simulink model "DCmotormodelREF"  (R2024b)
settings: Solver=VariableStepAuto  StartTime=0.0  StopTime=18  MaxStep=1e-4  RelTol=1e-4  AbsTol=1e-5
values from neighbouring files (symbols this model uses):
  Ctot = TMa/10 + 0.072 + Jmotor * omega_max_rad/ta    (= 0.152406290556)    [DCMOTORELAST.m]    (also in simulazione_vuota1.mat = 0.152406290545; simulazione_vuota2lim.mat = 0.152406290545)
  ilim = 1*Ia_nom    (= 3.65)    [DCMOTORELAST.m]    (also in simulazione_vuota1.mat = 4.38; simulazione_vuota2lim.mat = 4.38)
  Jtot = (Ctot*ta) / omega_max_rad    (= 0.000727686435009)    [DCMOTORELAST.m]    (also in simulazione_vuota1.mat = 0.000727686435787; simulazione_vuota2lim.mat = 0.000727686435787)
  kamp = Va_lim/dcvolt    (= 5.76)    [DCMOTORELAST.m]    (also in simulazione_vuota1.mat; simulazione_vuota2lim.mat)
  kdt = Vctr/omega_max_rad    (= 0.0131293711322)    [DCMOTORELAST.m]    (also in simulazione_vuota1.mat = 0.0131278037994; simulazione_vuota2lim.mat = 0.0131278037994)
  kff = kv/(kamp*kdt)    (= 0.921781173607)    [DCMOTORELAST.m]
  ki = Ki_opt    (= 56)    [DCMOTORELAST.m]
  klim_corr = dcvolt/(0.2*Ia_nom)    (= 6.84931506849)    [DCMOTORELAST.m]    (also in simulazione_vuota1.mat; simulazione_vuota2lim.mat)
  kp = kpf    [DCMOTORELAST.m]
  Kpos = Kpos_vec(ii)    [DCMOTORELAST.m]
  kt = kv    (= 0.0697098650743)    [DCMOTORELAST.m]    (also in simulazione_vuota1.mat = 0.0697; simulazione_vuota2lim.mat = 0.0697)
  kv = kvC*60/(1000*2*pi)    (= 0.0697098650743)    [DCMOTORELAST.m]    (also in simulazione_vuota1.mat = 0.0697; simulazione_vuota2lim.mat = 0.0697)
  S_wu = 1.2*(Ra*Iamax/kamp)    (= 0.387156307417)    [DCMOTORELAST.m]
  Va_lim = 1.2*Va_nom    (= 28.8)    [DCMOTORELAST.m]    (also in simulazione_vuota1.mat; simulazione_vuota2lim.mat)
  Vctr = Va/kamp    (= 4.12471358951)    [DCMOTORELAST.m]    (also in simulazione_vuota1.mat = 4.12422119268; simulazione_vuota2lim.mat = 4.12422119268)
libraries: cstblocks x2
settings Model: Creator=marco  LastModifiedBy=david

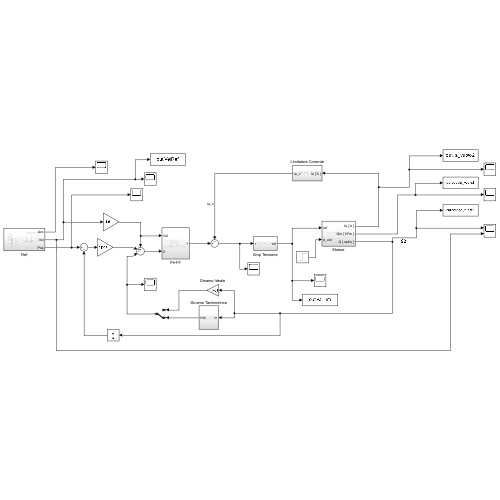
[thumbnail: Simulink's stored preview of the top-level diagram]
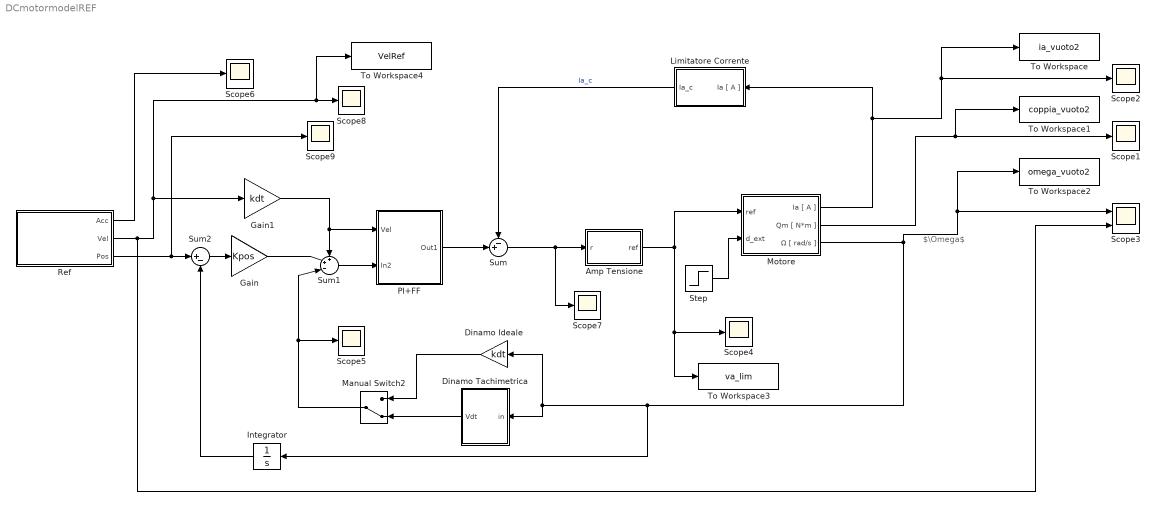
== system DCmotormodelREF ==
  note: $\Omega$
  Amp Tensione : Subsystem
  Dinamo Ideale : Gain  Gain=kdt
  Dinamo Tachimetrica : Subsystem
  Gain : Gain  Gain=Kpos
  Gain1 : Gain  Gain=kdt
  Integrator : Integrator
  Limitatore Corrente : Subsystem
  Manual Switch2 : ManualSwitch  CurrentSetting=0
  Motore : Subsystem
  PI+FF : Subsystem
  Ref : Subsystem
  Scope{1..2,4..9} (8 alike) : Scope
  Scope3 : Scope  NumInputPorts=2
  Step : Step  Time=5  After=Vctr*0.8*0.01  SampleTime=0
  Sum : Sum  Inputs=-+|
  Sum1 : Sum  Inputs=++-|
  Sum2 : Sum  Inputs=|+-
  To Workspace : ToWorkspace  VariableName=ia_vuoto2  SaveFormat=Timeseries  SampleTime=-1
  To Workspace1 : ToWorkspace  VariableName=coppia_vuoto2  SaveFormat=Timeseries  SampleTime=-1
  To Workspace2 : ToWorkspace  VariableName=omega_vuoto2  SaveFormat=Timeseries  SampleTime=-1
  To Workspace3 : ToWorkspace  VariableName=va_lim  SaveFormat=Timeseries  SampleTime=-1
  To Workspace4 : ToWorkspace  VariableName=VelRef  SaveFormat=Timeseries  SampleTime=-1
  wires:
  Motore/1(Ia [ A ]) -> Limitatore Corrente/1(Ia [ A ]), To Workspace/1, Scope2/1
  Motore/2(Qm [ N*m ]) -> To Workspace1/1, Scope1/1
  Motore/3(Ω [ rad/s ]) -> To Workspace2/1, Scope3/1, Integrator/1, Dinamo Tachimetrica/1(in), Dinamo Ideale/1
  Amp Tensione/1(ref) -> Motore/1(ref), Scope4/1, To Workspace3/1
  Sum/1 -> Amp Tensione/1(r), Scope7/1
  Limitatore Corrente/1(Ia_c) -> Sum/1  "Ia_c"
  Dinamo Tachimetrica/1(Vdt) -> Manual Switch2/2
  Manual Switch2/1 -> Scope5/1, Sum1/3
  Dinamo Ideale/1 -> Manual Switch2/1
  Sum1/1 -> PI+FF/2(In2)
  PI+FF/1(Out1) -> Sum/2
  Ref/1(Acc) -> Scope6/1
  Ref/2(Vel) -> Scope3/2, To Workspace4/1, Scope8/1, Gain1/1
  Ref/3(Pos) -> Sum2/1, Scope9/1
  Integrator/1 -> Sum2/2
  Sum2/1 -> Gain/1
  Gain/1 -> Sum1/2
  Gain1/1 -> Sum1/1, PI+FF/1(Vel)
  Step/1 -> Motore/2(d_ext)

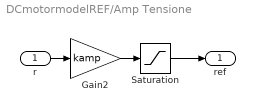
== system DCmotormodelREF/Amp Tensione ==
  r : Inport
  Gain2 : Gain  Gain=kamp
  Saturation : Saturate  UpperLimit=Va_lim  LowerLimit=-Va_lim
  ref : Outport
  wires:
  Saturation/1 -> ref/1
  Gain2/1 -> Saturation/1
  r/1 -> Gain2/1

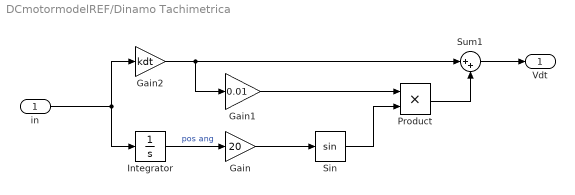
== system DCmotormodelREF/Dinamo Tachimetrica ==
  in : Inport
  Gain : Gain  Gain=20
  Gain1 : Gain  Gain=0.01
  Gain2 : Gain  Gain=kdt
  Integrator : Integrator
  Product : Product
  Sin : Trigonometry
  Sum1 : Sum  Inputs=|++
  Vdt : Outport
  wires:
  Integrator/1 -> Gain/1  "pos ang"
  Sum1/1 -> Vdt/1
  Gain/1 -> Sin/1
  Gain2/1 -> Gain1/1, Sum1/1
  Gain1/1 -> Product/1
  in/1 -> Integrator/1, Gain2/1
  Product/1 -> Sum1/2
  Sin/1 -> Product/2

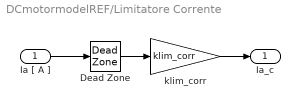
== system DCmotormodelREF/Limitatore Corrente ==
  Ia [ A ] : Inport
  Dead Zone : DeadZone  LowerValue=-ilim  UpperValue=ilim
  klim_corr : Gain  Gain=klim_corr
  Ia_c : Outport
  wires:
  Ia [ A ]/1 -> Dead Zone/1
  Dead Zone/1 -> klim_corr/1
  klim_corr/1 -> Ia_c/1

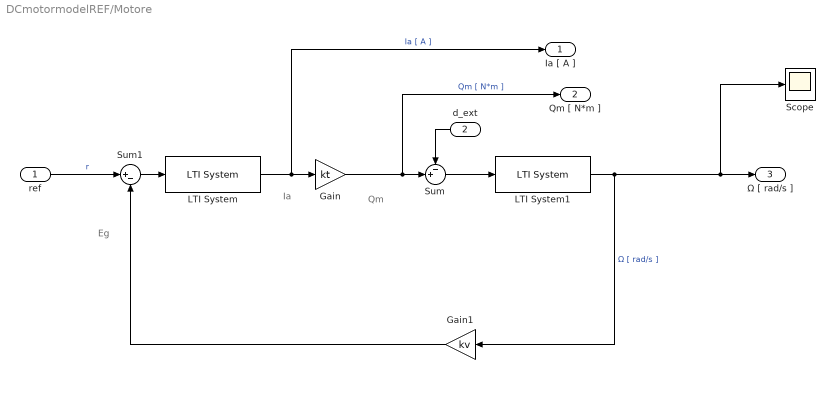
== system DCmotormodelREF/Motore ==
  note: Qm
  note: Ia
  note: Eg
  ref : Inport
  d_ext : Inport  Port=2
  Gain : Gain  Gain=kt
  Gain1 : Gain  Gain=kv
  LTI System : cstblocks/LTI System  sys=P_el  IC=[]  PadeOrder=0
  LTI System1 : cstblocks/LTI System  sys=P_mec  IC=[]  PadeOrder=0
  Scope : Scope
  Sum : Sum  Inputs=-+|
  Sum1 : Sum  Inputs=|+-
  Ia [ A ] : Outport
  Qm [ N*m ] : Outport  Port=2
  Ω [ rad/s ] : Outport  Port=3
  wires:
  Gain/1 -> Qm [ N*m ]/1, Sum/2  "Qm [ N*m ]"
  Sum/1 -> LTI System1/1
  Gain1/1 -> Sum1/2
  Sum1/1 -> LTI System/1
  LTI System1/1 -> Scope/1, Ω [ rad/s ]/1, Gain1/1  "Ω [ rad/s ]"
  LTI System/1 -> Ia [ A ]/1, Gain/1  "Ia [ A ]"
  ref/1 -> Sum1/1  "r"
  d_ext/1 -> Sum/1

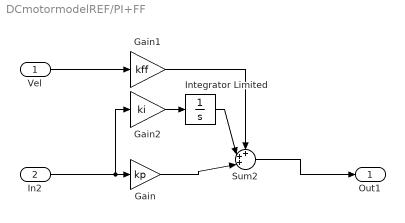
== system DCmotormodelREF/PI+FF ==
  Vel : Inport
  In2 : Inport  Port=2
  Gain : Gain  Gain=kp
  Gain1 : Gain  Gain=kff
  Gain2 : Gain  Gain=ki
  Integrator Limited : Integrator  LimitOutput=on  UpperSaturationLimit=S_wu  LowerSaturationLimit=-S_wu
  Sum2 : Sum  Inputs=+++|
  Out1 : Outport
  wires:
  Integrator Limited/1 -> Sum2/2
  Gain/1 -> Sum2/3
  In2/1 -> Gain2/1, Gain/1
  Vel/1 -> Gain1/1
  Gain2/1 -> Integrator Limited/1
  Gain1/1 -> Sum2/1
  Sum2/1 -> Out1/1

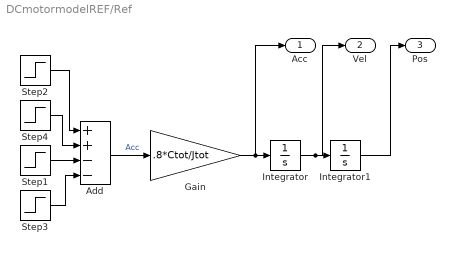
== system DCmotormodelREF/Ref ==
  Add : Sum  Inputs=++--
  Gain : Gain  Gain=.8*Ctot/Jtot
  Integrator : Integrator
  Integrator1 : Integrator
  Step1 : Step  Time=2.5  SampleTime=0
  Step2 : Step  SampleTime=0
  Step3 : Step  Time=14.5  SampleTime=0
  Step4 : Step  Time=16  SampleTime=0
  Acc : Outport
  Vel : Outport  Port=2
  Pos : Outport  Port=3
  wires:
  Step2/1 -> Add/1
  Step3/1 -> Add/4
  Integrator1/1 -> Pos/1
  Step1/1 -> Add/3
  Step4/1 -> Add/2
  Integrator/1 -> Vel/1, Integrator1/1
  Add/1 -> Gain/1  "Acc"
  Gain/1 -> Acc/1, Integrator/1
